simulink model "is_in_shadow_test"  (R2023b)
settings: Solver=VariableStepAuto  StartTime=0.0  StopTime=7200  RelTol=1e-3
libraries: vrlib x1
settings Model: Creator=laura  LastModifiedBy=laura

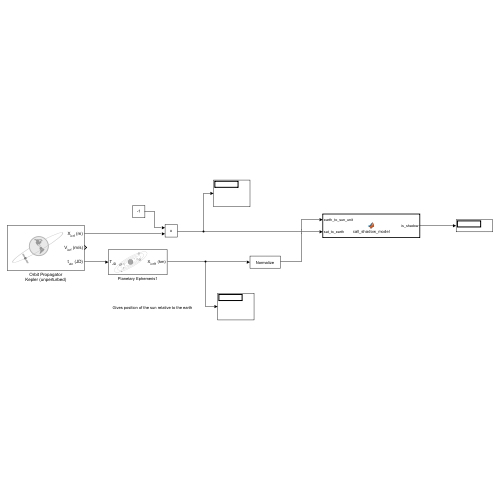
[thumbnail: Simulink's stored preview of the top-level diagram]
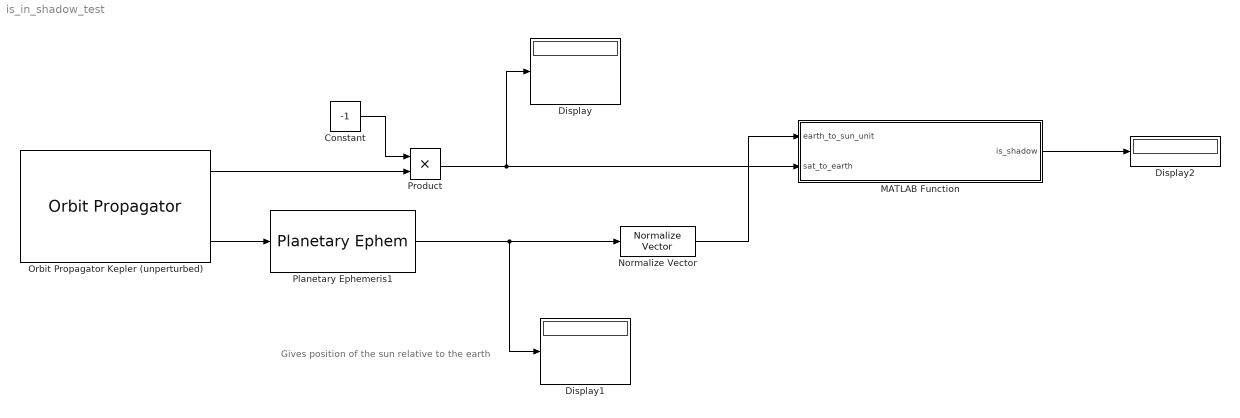
== system is_in_shadow_test ==
  note: Gives position of the sun relative to the earth
  Constant : Constant  Value=-1
  Display : Display
  Display1 : Display
  Display2 : Display
  MATLAB Function : MATLAB Function  TreatAsAtomicUnit=on
  Normalize Vector : vrlib/Utilities/Normalize Vector  maxzero=0
  Orbit Propagator Kepler (unperturbed) : OrbitPropagator  inertialPosition=[3649700.0 3308200.0 -4676600.0]  inertialVelocity=[-2750.8 6666.4 2573.4]  fixedPosition=[-4142689.0 -2676864.7 -4669861.6]  fixedVelocity=[1452.7 -6720.7 2568.1]  customR=3396200  customMu=4.305e13  customJ2=1.0826269e-03  customOmega=4.06125949e-3
  Planetary Ephemeris1 : PlanetaryEphem  target=Sun  outputVelocity=off
  Product : Product
  wires:
  Orbit Propagator Kepler (unperturbed)/3 -> Planetary Ephemeris1/1
  Orbit Propagator Kepler (unperturbed)/1 -> Product/2
  Planetary Ephemeris1/1 -> Display1/1, Normalize Vector/1
  Normalize Vector/1 -> MATLAB Function/1(earth_to_sun_unit)
  MATLAB Function/1(is_shadow) -> Display2/1
  Product/1 -> Display/1, MATLAB Function/2(sat_to_earth)
  Constant/1 -> Product/1

== matlab function is_in_shadow_test/MATLAB Function ==
  data: earth_to_sun_unit input; is_shadow output; sat_to_earth input
function is_shadow = call_shadow_model(earth_to_sun_unit,sat_to_earth)

is_shadow = is_in_shadow(earth_to_sun_unit,sat_to_earth);
